simulink model "fullsystem"  (Simulink 8.5)
settings: Solver=ode15s  SolverMode=SingleTasking  StartTime=0.0  StopTime=0.1  RelTol=1e-3  AbsTol=1e-6
undefined symbols (not defined in the file or in its folder): DAB, den, elements, num
libraries: powerlib x43, powerlib_extras x1
(part 1 of 6)
settings Model: Creator=Dr. Lotfifard  LastModifiedBy=PC  ExtModeTrigMode=oneshot  ExtModeArmWhenConnect=off
settings SolverCC: ZeroCrossAlgorithm=Adaptive
settings DataIOCC: LimitDataPoints=off
settings OptimizationCC: BlockReduction=off  BooleanDataType=off
settings DebuggingCC: SaveWithParameterizedLinksMsg=none  SignalResolutionControl=TryResolveAllWithWarning  MultiTaskDSMMsg=warning  MultiTaskCondExecSysMsg=none  FcnCallInpInsideContextMsg=UseLocalSettings
settings HardwareCC: TargetUnknown=on

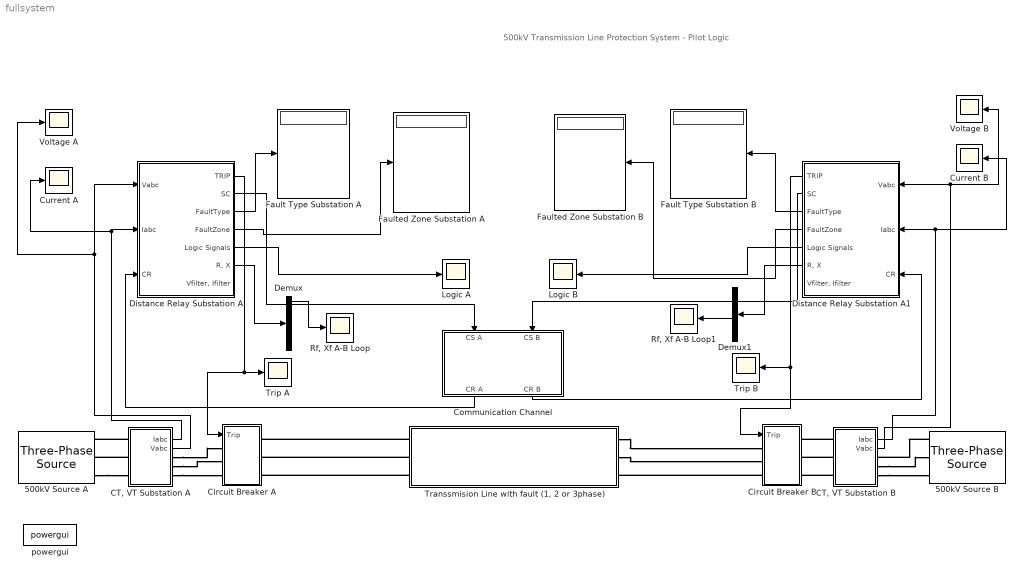
== system fullsystem ==
  note: 500kV Transmission Line Protection System - Pilot Logic
  500kV Source A : powerlib/Electrical Sources/Three-Phase Source  Voltage=500000/sqrt(3)*sqrt(2)  PhaseAngle=0  Frequency=60  InternalConnection=Yg  SpecifyImpedance=off  Resistance=0.724  Inductance=19.2e-3  ShortCircuitLevel=100e6  BaseVoltage=25e3  XRratio=7  BusType=swing  Pref=0  Qref=0  Qmin=-inf  Qmax=inf
  500kV Source B : powerlib/Electrical Sources/Three-Phase Source  Voltage=1.05*500000/sqrt(3)*sqrt(2)  PhaseAngle=10  Frequency=60  InternalConnection=Yg  SpecifyImpedance=off  Resistance=0.724  Inductance=19.2e-3  ShortCircuitLevel=100e6  BaseVoltage=25e3  XRratio=7  BusType=swing  Pref=0  Qref=0  Qmin=-inf  Qmax=inf
  "CT, VT Substation A" : Subsystem  mask{VT=1, CT=1}
      mask prompts: VT "VT ratio"; CT "CT ratio"
  "CT, VT Substation B" : Subsystem  mask{VT=1, CT=1}
      mask prompts: VT "VT ratio"; CT "CT ratio"
  Circuit Breaker A : Subsystem
  Circuit Breaker B : Subsystem
  Communication Channel : Subsystem  mask(Communication channel.){Tdelay=0, failureA=on, failureB=on, err_signal=0}
      mask prompts: Tdelay "Channel delay time [ms]:"; failureA "A to B Communication channel failure."; failureB "B to A Communication Channel failure"; err_signal "Erroneous signal:"
      mask TypeOptions err_signal: 0 | 1
  Current A : Scope
      settings: TickLabels=on  YMin=-8000  YMax=9000
  Current B : Scope
      settings: TickLabels=on  YMin=-8000  YMax=9000  SaveName=ScopeData2
  Demux : Demux  Outputs=6
  Demux1 : Demux  Outputs=6
  Distance Relay Substation A : Subsystem  mask{ZoneImpedance=[90 115 200 250 50], ZoneTime=[0 0.33 1 0.33 0.66], k0m1=0.726, k0a1=-3.69, LineAngle=84, Zstarter=300, Tstarter=0, underV=0.8*500000/sqrt(3)*sqrt(2), PilotLogic='PUTT', fCut=180, fSampling=24*60, WindowSize=24, VoltageRange=480, CurrentRange=480}
      mask prompts: ZoneImpedance "Zone Impedances [Z1 Z2 Z3 Z4 ZR] (Ohm):"; ZoneTime "Zone Times [T1 T2 T3 T4 TR] (s):"; LineAngle "Line Angle:"; Zstarter "Starter Impedance (Ohm):"; Tstarter "Starter Time (s):"; underV "UnderVoltage Threshold (V):"; PilotLogic "Pilot Logic Scheme:"; fCut "fCut (Hz):"; fSampling "fSampling (Hz):"; WindowSize "Window Size (samples):"; VoltageRange "Voltage Range (V):"; CurrentRange "Current Range (A):"
      mask TypeOptions PilotLogic: 'BLOV+TB' | 'PUTT'
  Distance Relay Substation A1 : Subsystem  mask{ZoneImpedance=[90 115 200 250 50], ZoneTime=[0 0.33 1 0.33 0.66], k0m1=0.726, k0a1=-3.69, LineAngle=84, Zstarter=300, Tstarter=0, underV=0.8*1.05*500000/sqrt(3)*sqrt(2), PilotLogic='PUTT', fCut=180, fSampling=24*60, WindowSize=24, VoltageRange=480, CurrentRange=480}
      mask prompts: ZoneImpedance "Zone Impedances [Z1 Z2 Z3 Z4 ZR] (Ohm):"; ZoneTime "Zone Times [T1 T2 T3 T4 TR] (s):"; LineAngle "Line Angle:"; Zstarter "Starter Impedance (Ohm):"; Tstarter "Starter Time (s):"; underV "UnderVoltage Threshold (V):"; PilotLogic "Pilot Logic Scheme:"; fCut "fCut (Hz):"; fSampling "fSampling (Hz):"; WindowSize "Window Size (samples):"; VoltageRange "Voltage Range (V):"; CurrentRange "Current Range (A):"
      mask TypeOptions PilotLogic: 'BLOV+TB' | 'PUTT'
  Fault Type Substation A : Display
  Fault Type Substation B : Display
  Faulted Zone Substation A : Display
  Faulted Zone Substation B : Display
  Logic A : Scope
      settings: SaveName=ScopeData5
  Logic B : Scope
      settings: SaveName=ScopeData4
  "Rf, Xf A-B Loop" : Scope
      settings: YMin=-450  YMax=125
  "Rf, Xf A-B Loop1" : Scope
      settings: SaveName=ScopeData6
  "Transsmision Line with fault (1, 2 or 3phase)" : Subsystem  mask(Teansmission line with fault){ff=60, rr=[0.025485 0.57504], ll=[1.5760e-3 4.5291e-3], cc=[19.1e-9 11.2e-9], length=200, faultLocation=0.5, faultType='A-G', faultR=0.1, faultTime=[0.034 1 2 3 4]}
      mask prompts: ff "Frequency used for R L C specification (Hz)"; rr "Resistance per unit length (Ohm/km) [R1 R0]"; ll "Inductance per unit length (H/km) [L1 L0]"; cc "Capacitance per unit length (F/km) [C1 C0]"; length "Line length (km)"; faultLocation "Fault location (p.u.) <0,1>"; faultType "Fault Type"; faultR "Fault Resistance per Phase (Ohm)"; faultTime "Fault time sequence (s) [C O C O C]"
      mask TypeOptions faultType: 'A-G' | 'A-B' | 'A-B-G' | 'A-B-C' | 'A-B-C-G'
  Trip A : Scope
      settings: SaveName=ScopeData3
  Trip B : Scope
      settings: SaveName=ScopeData7
  Voltage A : Scope
      settings: TickLabels=on  YMin=-400000  YMax=400000
  Voltage B : Scope
      settings: TickLabels=on  SaveName=ScopeData8
  powergui : powerlib/powergui  SimulationMode=Continuous  SolverType=Tustin/Backward Euler (TBE)  SampleTime=0  frequency=60  SPID=off  DisableSnubberDevices=off  DisableRonSwitches=off  DisableVfSwitches=off  SwTol=0  DisplayEquations=off  Interpol=off  methode=off  Ts=0  FunctionMessages=off  echomessages=off  HookPort=off  EnableUseOfTLC=off  x0status=blocks  frequencyindice=60  Pbase=100e6  ErrMax=1e-4  Iterations=50  UnitsV=kV  UnitsW=MW  buscounter=0  RestoreLinks=warning  ResistiveCurrentMeasurement=off  Frange=[0:2:500]  Ylog=off  Xlog=on  ShowGrid=off  save=off  variable=ZData  structure=0  ZoomFFT=on  StartTime=0.0  cycles=1  DisplayStyle=1  fundamental=60  FreqAxis=off  MaxFrequency=1000  frequencyindicesteady=1  RmsSteady=1  display=off
  wires:
  "CT, VT Substation A"/2(Vabc) -> Voltage A/1, Distance Relay Substation A/1(Vabc)
  "CT, VT Substation A"/1(Iabc) -> Current A/1, Distance Relay Substation A/2(Iabc)
  Distance Relay Substation A/3(FaultType) -> Fault Type Substation A/1
  Distance Relay Substation A/4(FaultZone) -> Faulted Zone Substation A/1
  Distance Relay Substation A/1("TRIP ") -> Circuit Breaker A/1(Trip), Trip A/1
  Distance Relay Substation A/5(Logic Signals) -> Logic A/1
  Distance Relay Substation A/6("R, X") -> Demux/1
  Distance Relay Substation A1/3(FaultType) -> Fault Type Substation B/1
  Distance Relay Substation A1/4(FaultZone) -> Faulted Zone Substation B/1
  Distance Relay Substation A1/1("TRIP ") -> Circuit Breaker B/1(Trip), Trip B/1
  Distance Relay Substation A1/6("R, X") -> Demux1/1
  Demux1/4 -> "Rf, Xf A-B Loop1"/1
  Distance Relay Substation A1/5(Logic Signals) -> Logic B/1
  "CT, VT Substation B"/1(Iabc) -> Distance Relay Substation A1/2(Iabc), Current B/1
  "CT, VT Substation B"/2(Vabc) -> Distance Relay Substation A1/1(Vabc), Voltage B/1
  Communication Channel/2(CR B) -> Distance Relay Substation A1/3(CR)
  Distance Relay Substation A1/2(SC) -> Communication Channel/2(CS B)
  Distance Relay Substation A/2(SC) -> Communication Channel/1(CS A)
  Communication Channel/1(CR A) -> Distance Relay Substation A/3(CR)
  Demux/1 -> "Rf, Xf A-B Loop"/1
  connections:
  "CT, VT Substation A"/LConn1 -- 500kV Source A/RConn1
  500kV Source A/RConn3 -- "CT, VT Substation A"/LConn3
  "CT, VT Substation A"/LConn2 -- 500kV Source A/RConn2
  "CT, VT Substation A"/RConn3 -- Circuit Breaker A/LConn3
  "Transsmision Line with fault (1, 2 or 3phase)"/LConn1 -- Circuit Breaker A/RConn1
  "Transsmision Line with fault (1, 2 or 3phase)"/LConn2 -- Circuit Breaker A/RConn2
  "Transsmision Line with fault (1, 2 or 3phase)"/LConn3 -- Circuit Breaker A/RConn3
  Circuit Breaker B/LConn3 -- "Transsmision Line with fault (1, 2 or 3phase)"/RConn3
  "Transsmision Line with fault (1, 2 or 3phase)"/RConn2 -- Circuit Breaker B/LConn2
  "Transsmision Line with fault (1, 2 or 3phase)"/RConn1 -- Circuit Breaker B/LConn1
  "CT, VT Substation B"/LConn1 -- Circuit Breaker B/RConn1
  "CT, VT Substation B"/LConn2 -- Circuit Breaker B/RConn2
  "CT, VT Substation B"/LConn3 -- Circuit Breaker B/RConn3
  500kV Source B/RConn1 -- "CT, VT Substation B"/RConn1
  "CT, VT Substation B"/RConn2 -- 500kV Source B/RConn2
  "CT, VT Substation B"/RConn3 -- 500kV Source B/RConn3
  "CT, VT Substation A"/RConn1 -- Circuit Breaker A/LConn1
  "CT, VT Substation A"/RConn2 -- Circuit Breaker A/LConn2

== system fullsystem/CT, VT Substation A ==
  CT-ratio : Gain  Gain=1/CT  SaturateOnIntegerOverflow=on  OutDataTypeStr=Inherit: Same as input  ParamDataTypeStr=Inherit: Same as input
  Ground : powerlib/Elements/Ground  LConnTagsString=a
  IA : powerlib/Measurements/Current Measurement  PhasorSimulation=off  OutputType=Complex  PSBequivalent=0
  IB1 : powerlib/Measurements/Current Measurement  PhasorSimulation=off  OutputType=Complex  PSBequivalent=0
  IC1 : powerlib/Measurements/Current Measurement  PhasorSimulation=off  OutputType=Complex  PSBequivalent=0
  Mux : Mux  Inputs=3
  Mux1 : Mux  Inputs=3
  VA1 : powerlib/Measurements/Voltage Measurement  PhasorSimulation=off  OutputType=Complex  PSBequivalent=0
  VB1 : powerlib/Measurements/Voltage Measurement  PhasorSimulation=off  OutputType=Complex  PSBequivalent=0
  VC1 : powerlib/Measurements/Voltage Measurement  PhasorSimulation=off  OutputType=Complex  PSBequivalent=0
  VT-ratio : Gain  Gain=1/VT  SaturateOnIntegerOverflow=on  OutDataTypeStr=Inherit: Same as input  ParamDataTypeStr=Inherit: Same as input
  Ain : PMIOPort  Port=1  Side=Left
  Bin : PMIOPort  Port=2  Side=Left
  Cin : PMIOPort  Port=3  Side=Left
  Aout : PMIOPort  Port=4  Side=Right
  Bout : PMIOPort  Port=5  Side=Right
  Cout : PMIOPort  Port=6  Side=Right
  Iabc : Outport
  Vabc : Outport  Port=2
  wires:
  Mux/1 -> CT-ratio/1
  Mux1/1 -> VT-ratio/1
  IA/1 -> Mux/1
  IB1/1 -> Mux/2
  IC1/1 -> Mux/3
  VC1/1 -> Mux1/3
  VB1/1 -> Mux1/2
  VA1/1 -> Mux1/1
  CT-ratio/1 -> Iabc/1
  VT-ratio/1 -> Vabc/1
  connections:
  VC1/LConn2 -- Ground/LConn1 -- VB1/LConn2 -- VA1/LConn2
  Ain/RConn1 -- IA/LConn1 -- VA1/LConn1
  IB1/LConn1 -- Bin/RConn1 -- VB1/LConn1
  IC1/LConn1 -- Cin/RConn1 -- VC1/LConn1
  Cout/RConn1 -- IC1/RConn1
  Aout/RConn1 -- IA/RConn1
  Bout/RConn1 -- IB1/RConn1

== system fullsystem/CT, VT Substation B ==
  CT-ratio : Gain  Gain=1/CT  SaturateOnIntegerOverflow=on  OutDataTypeStr=Inherit: Same as input  ParamDataTypeStr=Inherit: Same as input
  Ground : powerlib/Elements/Ground  LConnTagsString=a
  IA : powerlib/Measurements/Current Measurement  PhasorSimulation=off  OutputType=Complex  PSBequivalent=0
  IB1 : powerlib/Measurements/Current Measurement  PhasorSimulation=off  OutputType=Complex  PSBequivalent=0
  IC1 : powerlib/Measurements/Current Measurement  PhasorSimulation=off  OutputType=Complex  PSBequivalent=0
  Mux : Mux  Inputs=3
  Mux1 : Mux  Inputs=3
  VA1 : powerlib/Measurements/Voltage Measurement  PhasorSimulation=off  OutputType=Complex  PSBequivalent=0
  VB1 : powerlib/Measurements/Voltage Measurement  PhasorSimulation=off  OutputType=Complex  PSBequivalent=0
  VC1 : powerlib/Measurements/Voltage Measurement  PhasorSimulation=off  OutputType=Complex  PSBequivalent=0
  VT-ratio : Gain  Gain=1/VT  SaturateOnIntegerOverflow=on  OutDataTypeStr=Inherit: Same as input  ParamDataTypeStr=Inherit: Same as input
  Ain : PMIOPort  Port=1  Side=Left
  Bin : PMIOPort  Port=2  Side=Left
  Cin : PMIOPort  Port=3  Side=Left
  Aout : PMIOPort  Port=4  Side=Right
  Bout : PMIOPort  Port=5  Side=Right
  Cout : PMIOPort  Port=6  Side=Right
  Iabc : Outport
  Vabc : Outport  Port=2
  wires:
  Mux/1 -> CT-ratio/1
  Mux1/1 -> VT-ratio/1
  IA/1 -> Mux/1
  IB1/1 -> Mux/2
  IC1/1 -> Mux/3
  VC1/1 -> Mux1/3
  VB1/1 -> Mux1/2
  VA1/1 -> Mux1/1
  CT-ratio/1 -> Iabc/1
  VT-ratio/1 -> Vabc/1
  connections:
  VC1/LConn2 -- Ground/LConn1 -- VB1/LConn2 -- VA1/LConn2
  Ain/RConn1 -- IA/LConn1 -- VA1/LConn1
  IB1/LConn1 -- Bin/RConn1 -- VB1/LConn1
  IC1/LConn1 -- Cin/RConn1 -- VC1/LConn1
  Cout/RConn1 -- IC1/RConn1
  Aout/RConn1 -- IA/RConn1
  Bout/RConn1 -- IB1/RConn1

== system fullsystem/Circuit Breaker A ==
  Trip : Inport
  10000 ohms3 : powerlib/Elements/Series RLC Branch  LConnTagsString=__new0  RConnTagsString=__new0  BranchType=R  Resistance=10000  Inductance=1e-3  SetiL0=off  InitialCurrent=0  Capacitance=1e-6  Setx0=off  InitialVoltage=0  Measurements=None
  10000 ohms4 : powerlib/Elements/Series RLC Branch  LConnTagsString=__new0  RConnTagsString=__new0  BranchType=R  Resistance=10000  Inductance=1e-3  SetiL0=off  InitialCurrent=0  Capacitance=1e-6  Setx0=off  InitialVoltage=0  Measurements=None
  10000 ohms5 : powerlib/Elements/Series RLC Branch  LConnTagsString=__new0  RConnTagsString=__new0  BranchType=R  Resistance=10000  Inductance=1e-3  SetiL0=off  InitialCurrent=0  Capacitance=1e-6  Setx0=off  InitialVoltage=0  Measurements=None
  Breaker3 : powerlib/Elements/Breaker  InitialState=0  SwitchingTimes="[ 1/60  5/60 ]"  External=on  BreakerResistance=0.01  SnubberResistance=1e6  SnubberCapacitance=inf  Measurements=None  MoreParameters=off  NoBreakLoop=off
  Breaker4 : powerlib/Elements/Breaker  InitialState=0  SwitchingTimes="[ 1/60  5/60 ]"  External=on  BreakerResistance=0.01  SnubberResistance=1e6  SnubberCapacitance=inf  Measurements=None  MoreParameters=off  NoBreakLoop=off
  Breaker5 : powerlib/Elements/Breaker  InitialState=0  SwitchingTimes="[ 1/60  5/60 ]"  External=on  BreakerResistance=0.01  SnubberResistance=1e6  SnubberCapacitance=inf  Measurements=None  MoreParameters=off  NoBreakLoop=off
  NOT1 : Logic  Operator=NOT  Inputs=1
  Ain : PMIOPort  Port=1  Side=Left
  Aout : PMIOPort  Port=2  Side=Right
  Bin : PMIOPort  Port=3  Side=Right
  Bout : PMIOPort  Port=4  Side=Left
  Cin : PMIOPort  Port=5  Side=Left
  Cout : PMIOPort  Port=6  Side=Right
  wires:
  Trip/1 -> NOT1/1
  NOT1/1 -> Breaker3/1, Breaker4/1, Breaker5/1
  connections:
  10000 ohms3/LConn1 -- Ain/RConn1 -- Breaker3/LConn1
  Aout/RConn1 -- 10000 ohms3/RConn1 -- Breaker3/RConn1
  10000 ohms4/LConn1 -- Bin/RConn1 -- Breaker4/LConn1
  10000 ohms4/RConn1 -- Bout/RConn1 -- Breaker4/RConn1
  10000 ohms5/LConn1 -- Cin/RConn1 -- Breaker5/LConn1
  Cout/RConn1 -- 10000 ohms5/RConn1 -- Breaker5/RConn1

== system fullsystem/Circuit Breaker B ==
  Trip : Inport
  10000 ohms3 : powerlib/Elements/Series RLC Branch  LConnTagsString=__new0  RConnTagsString=__new0  BranchType=R  Resistance=10000  Inductance=1e-3  SetiL0=off  InitialCurrent=0  Capacitance=1e-6  Setx0=off  InitialVoltage=0  Measurements=None
  10000 ohms4 : powerlib/Elements/Series RLC Branch  LConnTagsString=__new0  RConnTagsString=__new0  BranchType=R  Resistance=10000  Inductance=1e-3  SetiL0=off  InitialCurrent=0  Capacitance=1e-6  Setx0=off  InitialVoltage=0  Measurements=None
  10000 ohms5 : powerlib/Elements/Series RLC Branch  LConnTagsString=__new0  RConnTagsString=__new0  BranchType=R  Resistance=10000  Inductance=1e-3  SetiL0=off  InitialCurrent=0  Capacitance=1e-6  Setx0=off  InitialVoltage=0  Measurements=None
  Breaker3 : powerlib/Elements/Breaker  InitialState=0  SwitchingTimes="[ 1/60  5/60 ]"  External=on  BreakerResistance=0.01  SnubberResistance=1e6  SnubberCapacitance=inf  Measurements=None  MoreParameters=off  NoBreakLoop=off
  Breaker4 : powerlib/Elements/Breaker  InitialState=0  SwitchingTimes="[ 1/60  5/60 ]"  External=on  BreakerResistance=0.01  SnubberResistance=1e6  SnubberCapacitance=inf  Measurements=None  MoreParameters=off  NoBreakLoop=off
  Breaker5 : powerlib/Elements/Breaker  InitialState=0  SwitchingTimes="[ 1/60  5/60 ]"  External=on  BreakerResistance=0.01  SnubberResistance=1e6  SnubberCapacitance=inf  Measurements=None  MoreParameters=off  NoBreakLoop=off
  NOT1 : Logic  Operator=NOT  Inputs=1
  Ain : PMIOPort  Port=1  Side=Left
  Aout : PMIOPort  Port=2  Side=Right
  Bin : PMIOPort  Port=3  Side=Right
  Bout : PMIOPort  Port=4  Side=Left
  Cin : PMIOPort  Port=5  Side=Left
  Cout : PMIOPort  Port=6  Side=Right
  wires:
  Trip/1 -> NOT1/1
  NOT1/1 -> Breaker3/1, Breaker4/1, Breaker5/1
  connections:
  10000 ohms3/LConn1 -- Ain/RConn1 -- Breaker3/LConn1
  Aout/RConn1 -- 10000 ohms3/RConn1 -- Breaker3/RConn1
  10000 ohms4/LConn1 -- Bin/RConn1 -- Breaker4/LConn1
  10000 ohms4/RConn1 -- Bout/RConn1 -- Breaker4/RConn1
  10000 ohms5/LConn1 -- Cin/RConn1 -- Breaker5/LConn1
  Cout/RConn1 -- 10000 ohms5/RConn1 -- Breaker5/RConn1

== system fullsystem/Communication Channel ==
  CS A : Inport
  CS B : Inport  Port=2
  " " : Constant  Value=failureA
  "  " : Constant  Value=err_signal-1
  " 1" : Constant  Value=failureB
  Switch : Switch  Threshold=0.5  SaturateOnIntegerOverflow=on  InputSameDT=on
  Switch1 : Switch  Threshold=0.5  SaturateOnIntegerOverflow=on  InputSameDT=on
  delay A->B : TransportDelay  DelayTime=Tdelay/1000+1e-12
  delay B->A : TransportDelay  DelayTime=Tdelay/1000+1e-12
  CR A : Outport  InitialOutput=0
  CR B : Outport  Port=2  InitialOutput=0
  wires:
  Switch/1 -> CR A/1
  CS B/1 -> delay A->B/1
  CS A/1 -> delay B->A/1
  Switch1/1 -> CR B/1
  "  "/1 -> Switch1/1, Switch/1
  delay A->B/1 -> Switch/3
  delay B->A/1 -> Switch1/3
  " "/1 -> Switch1/2
  " 1"/1 -> Switch/2

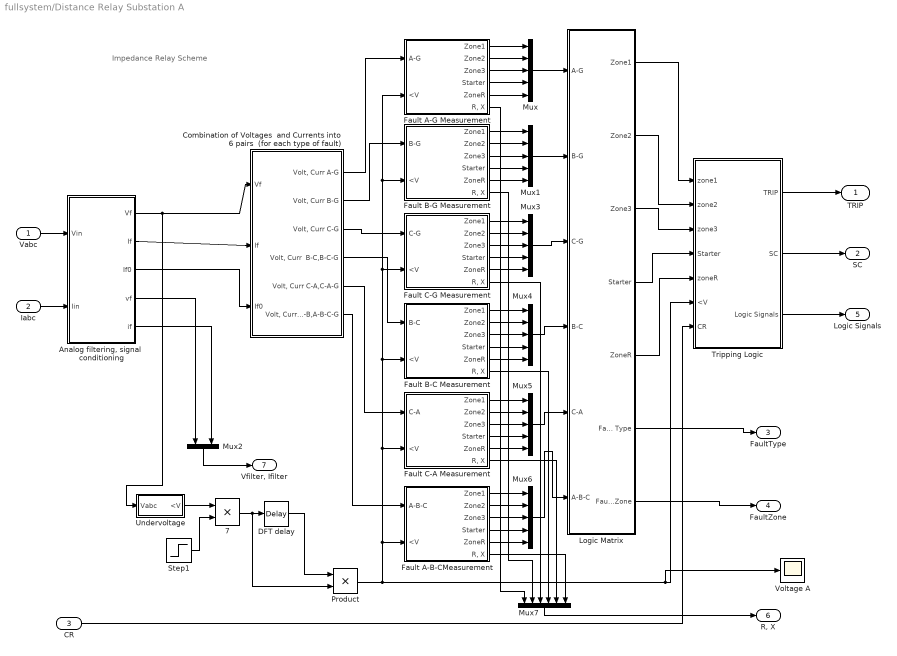
== system fullsystem/Distance Relay Substation A ==
  note: Impedance Relay Scheme
  Vabc : Inport
  Iabc : Inport  Port=2
  CR : Inport  Port=3
  " 7" : Product  RndMeth=Zero
  "Analog filtering, signal  conditioning" : Subsystem
  Combination of Voltages  and Currents into 6 pairs  (for each type of fault) : Subsystem
  DFT delay : TransportDelay  DelayTime=0.017  BufferSize=30720
  Fault A-B-CMeasurement : Subsystem
  Fault A-G Measurement : Subsystem
  Fault B-C Measurement : Subsystem
  Fault B-G Measurement : Subsystem
  Fault C-A Measurement : Subsystem
  Fault C-G Measurement : Subsystem
  Logic Matrix : Subsystem
  Mux{,1,3..6} (6 alike) : Mux  Inputs=5
  Mux2 : Mux  Inputs=2
  Mux7 : Mux  Inputs=6
  Product : Product  RndMeth=Zero
  Step1 : Step  Time=0.017  SampleTime=0
  Tripping Logic : Subsystem
  Undervoltage : Subsystem
  Voltage A : Scope
      settings: TickLabels=on  YMin=-400000  YMax=400000  SaveName=ScopeData9
  "TRIP " : Outport  InitialOutput=0
  SC : Outport  Port=2  InitialOutput=0
  FaultType : Outport  Port=3  InitialOutput=0
  FaultZone : Outport  Port=4  InitialOutput=0
  Logic Signals : Outport  Port=5  InitialOutput=0
  "R, X" : Outport  Port=6  InitialOutput=0
  "Vfilter, Ifilter" : Outport  Port=7  InitialOutput=0
  wires:
  Mux2/1 -> "Vfilter, Ifilter"/1
  Product/1 -> Fault A-B-CMeasurement/2(<V), Fault C-A Measurement/2(<V), Fault B-C Measurement/2(<V), Fault C-G Measurement/2(<V), Fault B-G Measurement/2(<V), Fault A-G Measurement/2(<V), Voltage A/1, Tripping Logic/6(<V)
  Logic Matrix/6(Fault Type) -> FaultType/1
  Tripping Logic/1(TRIP) -> "TRIP "/1
  Logic Matrix/3(" Zone3") -> Tripping Logic/3(zone3)
  Logic Matrix/2(" Zone2") -> Tripping Logic/2(zone2)
  Logic Matrix/1(" Zone1") -> Tripping Logic/1(zone1)
  Mux6/1 -> Logic Matrix/6(A-B-C)
  Mux5/1 -> Logic Matrix/5(C-A)
  Mux4/1 -> Logic Matrix/4(B-C)
  Mux3/1 -> Logic Matrix/3(C-G)
  Mux1/1 -> Logic Matrix/2(B-G)
  Mux/1 -> Logic Matrix/1(A-G)
  Fault B-G Measurement/2(Zone2) -> Mux1/2
  Fault A-G Measurement/4(Starter) -> Mux/4
  Fault A-G Measurement/3(Zone3) -> Mux/3
  Fault A-G Measurement/2(Zone2) -> Mux/2
  Fault A-G Measurement/1(Zone1) -> Mux/1
  DFT delay/1 -> Product/1
  Combination of Voltages  and Currents into 6 pairs  (for each type of fault)/5("Volt, Curr C-A,C-A-G") -> Fault C-A Measurement/1(C-A)
  Combination of Voltages  and Currents into 6 pairs  (for each type of fault)/2("Volt, Curr B-G") -> Fault B-G Measurement/1(B-G)
  "Analog filtering, signal  conditioning"/3(If0) -> Combination of Voltages  and Currents into 6 pairs  (for each type of fault)/3(If0)
  "Analog filtering, signal  conditioning"/2(If) -> Combination of Voltages  and Currents into 6 pairs  (for each type of fault)/2(If)
  "Analog filtering, signal  conditioning"/5(if) -> Mux2/2
  "Analog filtering, signal  conditioning"/4(vf) -> Mux2/1
  "Analog filtering, signal  conditioning"/1(Vf) -> Undervoltage/1("Vabc  "), Combination of Voltages  and Currents into 6 pairs  (for each type of fault)/1(Vf)
  " 7"/1 -> Product/2, DFT delay/1
  Step1/1 -> " 7"/2
  Undervoltage/1(<V) -> " 7"/1
  Combination of Voltages  and Currents into 6 pairs  (for each type of fault)/1("Volt, Curr A-G") -> Fault A-G Measurement/1(A-G)
  Iabc/1 -> "Analog filtering, signal  conditioning"/2(Iin)
  Vabc/1 -> "Analog filtering, signal  conditioning"/1(Vin)
  Fault B-G Measurement/1(Zone1) -> Mux1/1
  Fault B-G Measurement/3(Zone3) -> Mux1/3
  Fault A-G Measurement/5(ZoneR) -> Mux/5
  Fault B-G Measurement/4(Starter) -> Mux1/4
  Fault B-G Measurement/5(ZoneR) -> Mux1/5
  Combination of Voltages  and Currents into 6 pairs  (for each type of fault)/3("Volt, Curr C-G") -> Fault C-G Measurement/1(C-G)
  Fault C-G Measurement/1(Zone1) -> Mux3/1
  Fault C-G Measurement/2(Zone2) -> Mux3/2
  Fault C-G Measurement/3(Zone3) -> Mux3/3
  Fault C-G Measurement/4(Starter) -> Mux3/4
  Fault C-G Measurement/5(ZoneR) -> Mux3/5
  Combination of Voltages  and Currents into 6 pairs  (for each type of fault)/4("Volt, Curr  B-C,B-C-G") -> Fault B-C Measurement/1(B-C)
  Fault B-C Measurement/1(Zone1) -> Mux4/1
  Fault B-C Measurement/2(Zone2) -> Mux4/2
  Fault B-C Measurement/3(Zone3) -> Mux4/3
  Fault B-C Measurement/4(Starter) -> Mux4/4
  Fault B-C Measurement/5(ZoneR) -> Mux4/5
  Fault C-A Measurement/1(Zone1) -> Mux5/1
  Fault C-A Measurement/2(Zone2) -> Mux5/2
  Fault C-A Measurement/3(Zone3) -> Mux5/3
  Fault C-A Measurement/4(Starter) -> Mux5/4
  Fault C-A Measurement/5(ZoneR) -> Mux5/5
  Fault A-B-CMeasurement/1(Zone1) -> Mux6/1
  Fault A-B-CMeasurement/2(Zone2) -> Mux6/2
  Fault A-B-CMeasurement/3(Zone3) -> Mux6/3
  Fault A-B-CMeasurement/4(Starter) -> Mux6/4
  Fault A-B-CMeasurement/5(ZoneR) -> Mux6/5
  Combination of Voltages  and Currents into 6 pairs  (for each type of fault)/6("Volt, Curr A-B,A-B-C-G") -> Fault A-B-CMeasurement/1(A-B-C)
  Mux7/1 -> "R, X"/1
  Fault A-B-CMeasurement/6("R, X") -> Mux7/6
  Fault C-A Measurement/6("R, X") -> Mux7/5
  Fault B-C Measurement/6("R, X") -> Mux7/4
  Fault C-G Measurement/6("R, X") -> Mux7/3
  Fault B-G Measurement/6("R, X") -> Mux7/2
  Fault A-G Measurement/6("R, X") -> Mux7/1
  Logic Matrix/7(Fault Zone) -> FaultZone/1
  Tripping Logic/2(SC) -> SC/1
  Tripping Logic/3(Logic Signals) -> Logic Signals/1
  CR/1 -> Tripping Logic/7(CR)
  Logic Matrix/4(" Starter") -> Tripping Logic/4(Starter)
  Logic Matrix/5(" ZoneR") -> Tripping Logic/5(zoneR)

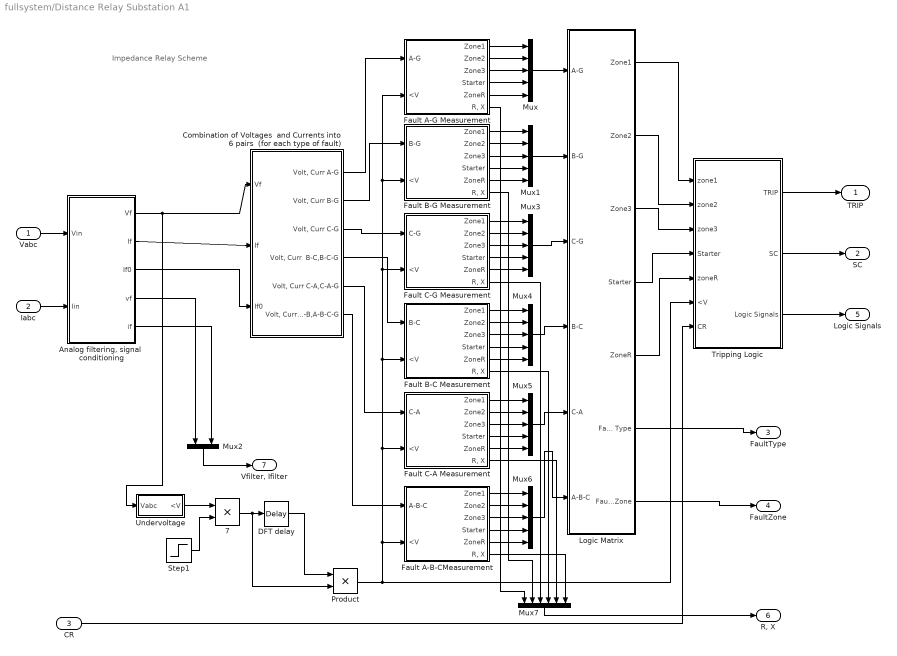
== system fullsystem/Distance Relay Substation A1 ==
  note: Impedance Relay Scheme
  Vabc : Inport
  Iabc : Inport  Port=2
  CR : Inport  Port=3
  " 7" : Product  RndMeth=Zero
  "Analog filtering, signal  conditioning" : Subsystem
  Combination of Voltages  and Currents into 6 pairs  (for each type of fault) : Subsystem
  DFT delay : TransportDelay  DelayTime=0.017  BufferSize=30720
  Fault A-B-CMeasurement : Subsystem
  Fault A-G Measurement : Subsystem
  Fault B-C Measurement : Subsystem
  Fault B-G Measurement : Subsystem
  Fault C-A Measurement : Subsystem
  Fault C-G Measurement : Subsystem
  Logic Matrix : Subsystem
  Mux{,1,3..6} (6 alike) : Mux  Inputs=5
  Mux2 : Mux  Inputs=2
  Mux7 : Mux  Inputs=6
  Product : Product  RndMeth=Zero
  Step1 : Step  Time=0.017  SampleTime=0
  Tripping Logic : Subsystem
  Undervoltage : Subsystem
  "TRIP " : Outport  InitialOutput=0
  SC : Outport  Port=2  InitialOutput=0
  FaultType : Outport  Port=3  InitialOutput=0
  FaultZone : Outport  Port=4  InitialOutput=0
  Logic Signals : Outport  Port=5  InitialOutput=0
  "R, X" : Outport  Port=6  InitialOutput=0
  "Vfilter, Ifilter" : Outport  Port=7  InitialOutput=0
  wires:
  Mux2/1 -> "Vfilter, Ifilter"/1
  Product/1 -> Fault A-B-CMeasurement/2(<V), Fault C-A Measurement/2(<V), Fault B-C Measurement/2(<V), Fault C-G Measurement/2(<V), Fault B-G Measurement/2(<V), Fault A-G Measurement/2(<V), Tripping Logic/6(<V)
  Logic Matrix/6(Fault Type) -> FaultType/1
  Tripping Logic/1(TRIP) -> "TRIP "/1
  Logic Matrix/3(" Zone3") -> Tripping Logic/3(zone3)
  Logic Matrix/2(" Zone2") -> Tripping Logic/2(zone2)
  Logic Matrix/1(" Zone1") -> Tripping Logic/1(zone1)
  Mux6/1 -> Logic Matrix/6(A-B-C)
  Mux5/1 -> Logic Matrix/5(C-A)
  Mux4/1 -> Logic Matrix/4(B-C)
  Mux3/1 -> Logic Matrix/3(C-G)
  Mux1/1 -> Logic Matrix/2(B-G)
  Mux/1 -> Logic Matrix/1(A-G)
  Fault B-G Measurement/2(Zone2) -> Mux1/2
  Fault A-G Measurement/4(Starter) -> Mux/4
  Fault A-G Measurement/3(Zone3) -> Mux/3
  Fault A-G Measurement/2(Zone2) -> Mux/2
  Fault A-G Measurement/1(Zone1) -> Mux/1
  DFT delay/1 -> Product/1
  Combination of Voltages  and Currents into 6 pairs  (for each type of fault)/5("Volt, Curr C-A,C-A-G") -> Fault C-A Measurement/1(C-A)
  Combination of Voltages  and Currents into 6 pairs  (for each type of fault)/2("Volt, Curr B-G") -> Fault B-G Measurement/1(B-G)
  "Analog filtering, signal  conditioning"/3(If0) -> Combination of Voltages  and Currents into 6 pairs  (for each type of fault)/3(If0)
  "Analog filtering, signal  conditioning"/2(If) -> Combination of Voltages  and Currents into 6 pairs  (for each type of fault)/2(If)
  "Analog filtering, signal  conditioning"/5(if) -> Mux2/2
  "Analog filtering, signal  conditioning"/4(vf) -> Mux2/1
  "Analog filtering, signal  conditioning"/1(Vf) -> Undervoltage/1("Vabc  "), Combination of Voltages  and Currents into 6 pairs  (for each type of fault)/1(Vf)
  " 7"/1 -> Product/2, DFT delay/1
  Step1/1 -> " 7"/2
  Undervoltage/1(<V) -> " 7"/1
  Combination of Voltages  and Currents into 6 pairs  (for each type of fault)/1("Volt, Curr A-G") -> Fault A-G Measurement/1(A-G)
  Iabc/1 -> "Analog filtering, signal  conditioning"/2(Iin)
  Vabc/1 -> "Analog filtering, signal  conditioning"/1(Vin)
  Fault B-G Measurement/1(Zone1) -> Mux1/1
  Fault B-G Measurement/3(Zone3) -> Mux1/3
  Fault A-G Measurement/5(ZoneR) -> Mux/5
  Fault B-G Measurement/4(Starter) -> Mux1/4
  Fault B-G Measurement/5(ZoneR) -> Mux1/5
  Combination of Voltages  and Currents into 6 pairs  (for each type of fault)/3("Volt, Curr C-G") -> Fault C-G Measurement/1(C-G)
  Fault C-G Measurement/1(Zone1) -> Mux3/1
  Fault C-G Measurement/2(Zone2) -> Mux3/2
  Fault C-G Measurement/3(Zone3) -> Mux3/3
  Fault C-G Measurement/4(Starter) -> Mux3/4
  Fault C-G Measurement/5(ZoneR) -> Mux3/5
  Combination of Voltages  and Currents into 6 pairs  (for each type of fault)/4("Volt, Curr  B-C,B-C-G") -> Fault B-C Measurement/1(B-C)
  Fault B-C Measurement/1(Zone1) -> Mux4/1
  Fault B-C Measurement/2(Zone2) -> Mux4/2
  Fault B-C Measurement/3(Zone3) -> Mux4/3
  Fault B-C Measurement/4(Starter) -> Mux4/4
  Fault B-C Measurement/5(ZoneR) -> Mux4/5
  Fault C-A Measurement/1(Zone1) -> Mux5/1
  Fault C-A Measurement/2(Zone2) -> Mux5/2
  Fault C-A Measurement/3(Zone3) -> Mux5/3
  Fault C-A Measurement/4(Starter) -> Mux5/4
  Fault C-A Measurement/5(ZoneR) -> Mux5/5
  Fault A-B-CMeasurement/1(Zone1) -> Mux6/1
  Fault A-B-CMeasurement/2(Zone2) -> Mux6/2
  Fault A-B-CMeasurement/3(Zone3) -> Mux6/3
  Fault A-B-CMeasurement/4(Starter) -> Mux6/4
  Fault A-B-CMeasurement/5(ZoneR) -> Mux6/5
  Combination of Voltages  and Currents into 6 pairs  (for each type of fault)/6("Volt, Curr A-B,A-B-C-G") -> Fault A-B-CMeasurement/1(A-B-C)
  Mux7/1 -> "R, X"/1
  Fault A-B-CMeasurement/6("R, X") -> Mux7/6
  Fault C-A Measurement/6("R, X") -> Mux7/5
  Fault B-C Measurement/6("R, X") -> Mux7/4
  Fault C-G Measurement/6("R, X") -> Mux7/3
  Fault B-G Measurement/6("R, X") -> Mux7/2
  Fault A-G Measurement/6("R, X") -> Mux7/1
  Logic Matrix/7(Fault Zone) -> FaultZone/1
  Tripping Logic/2(SC) -> SC/1
  Tripping Logic/3(Logic Signals) -> Logic Signals/1
  CR/1 -> Tripping Logic/7(CR)
  Logic Matrix/4(" Starter") -> Tripping Logic/4(Starter)
  Logic Matrix/5(" ZoneR") -> Tripping Logic/5(zoneR)

== system fullsystem/Transsmision Line with fault (1, 2 or 3phase) ==
  Fault Selector : Subsystem
  Fault1 : Subsystem
  Line1 : powerlib/Elements/Distributed Parameters Line  Phases=3  Frequency=ff  Resistance=rr  Inductance=ll  Capacitance=cc  Length=length*(faultLocation+0.0005)  x1=[0 1.53266796670346e-009 -40255.985134743 -39683.0380465592;2.86312968195295e-005 1.53189939694959e-009 -39825.3198862797 -40115.2308198371;5.7262593639059e-005 1.53095235510765e-009 -39390.0148370482 -40542.7500166237;8.58938904585885e-005 1.52982695151157e-009 -38950.120701737 -40965.5458293116;0.000114525187278118 1.52852331727516e-009 -38505.688729681 -41383.5690005856;0.000143156484097647 1.52704160427675e-009 -38056.77069889 -41796.7708291612]  x2=[0 1.55925131848491e-009 -40620.0878760363 -39910.0233219334;2.86312968195295e-005 1.55881129165316e-009 -40186.9514443784 -40346.1328285791;5.7262593639059e-005 1.55818965739555e-009 -39749.1330805045 -40777.5418577741;8.58938904585885e-005 1.55738648813482e-009 -39306.6837919141 -41204.2001487306;0.000114525187278118 1.55640187744325e-009 -38859.6551256268 -41626.0579941401;0.000143156484097647 1.55523594003171e-009 -38408.0991621773 -42043.0662459641]  x3=[0 2.01885457122014e-012 -163.089263474603 -105.450555147554;2.86312968195295e-005 2.03239610658583e-012 -161.941578955542 -107.204722130146;5.7262593639059e-005 2.04570086009907e-012 -160.775027628515 -108.946399356132;8.58938904585885e-005 2.05876728170564e-012 -159.589745401176 -110.675383913513;0.000114525187278118 2.07159384911787e-012 -158.385870363398 -112.391474369031;0.000143156484097647 2.08417906799204e-012 -157.163542771187 -114.094470791643]  x4=[0 2.64131154335596e-012 -123.841881809461 -165.416317671308;2.86312968195295e-005 2.63470626197041e-012 -122.049240966749 -166.743373545949;5.7262593639059e-005 2.62779402731559e-012 -120.242380924704 -168.051003185349;8.58938904585885e-005 2.62057564469306e-012 -118.42151218937 -169.339054245695;0.000114525187278118 2.61305195507176e-012 -116.58684689886 -170.607376664157;0.000143156484097647 2.60522383499005e-012 -114.738598798635 -171.855822676363]  x5=0.000143156484097647  V1=[1.023e-09 5.653e+04 5.653e+04;377 377 377;-0.6096 -0.9539 -2.525]  V2=[1.009e-09 5.763e+04 5.763e+04;377 377 377;-0.5917 -0.9614 -2.532]  I1=[1.529e-12 193 193;377 377 377;-0.6847 -1.158 -2.729]  I2=[1.505e-12 205.7 205.7;377 377 377;-0.9069 -0.9704 -2.541]  nHarmo=1  Measurements=None
  Line2 : powerlib/Elements/Distributed Parameters Line  Phases=3  Frequency=ff  Resistance=rr  Inductance=ll  Capacitance=cc  Length=length*(1-faultLocation-0.0005)  x1=[0 1.43137261755031e-009 -51373.762200412 -24567.0115803634;0.000256257228747928 1.48443013216827e-009 -48764.5687185778 -29407.7938360784;0.000512514457495856 1.52364444798437e-009 -45700.6164679546 -33974.3308258324;0.000768771686243784 1.54864986805002e-009 -42210.4786357914 -38224.0368610064;0.00102502891499171 1.55921320186769e-009 -38326.7028447818 -42117.2808911256;0.00128128614373964 1.55523594003171e-009 -34085.5076270153 -45617.7560871077]  x2=[0 1.5552865834267e-009 -50810.114798948 -24266.9121672487;0.000256257228747928 1.62275226289842e-009 -48232.4960307204 -29054.7262706394;0.000512514457495856 1.67508480697045e-009 -45205.080389744 -33571.5876742822;0.000768771686243784 1.71179618336988e-009 -41756.1003375311 -37775.3739441089;0.00102502891499171 1.73254403655516e-009 -37917.719675861 -41626.8822589206;0.00128128614373964 1.73713488038629e-009 -33725.7336000921 -45090.195000142]  x3=[0 1.4523601474402e-012 -189.596238125285 -56.3258357388615;0.000256257228747928 1.62464711268222e-012 -183.279195992341 -74.3509892290754;0.000512514457495856 1.78178327191703e-012 -175.252965739737 -91.6827752763165;0.000768771686243784 1.92230323647857e-012 -165.592396764968 -108.159564609767;0.00102502891499171 2.04489657365404e-012 -154.387579651591 -123.627701314326;0.00128128614373964 2.14842002725272e-012 -141.743006020653 -137.942935763923]  x4=[0 2.19293673092143e-012 -193.598935066748 -45.2078125315412;0.000256257228747928 2.29222269793401e-012 -188.335634767859 -63.6708932672806;0.000512514457495856 2.37013231733818e-012 -181.315992033535 -81.540204842525;0.000768771686243784 2.42593903533621e-012 -172.605469230635 -98.64910523942;0.00102502891499171 2.45912242090544e-012 -162.285297193952 -114.838043729142;0.00128128614373964 2.46937301912888e-012 -150.451717700097 -129.956048777869]  x5=0.00128128614373964  V1=[1.009e-09 5.763e+04 5.763e+04;377 377 377;-0.5911 -0.961 -2.532]  V2=[1.016e-09 5.63e+04 5.63e+04;377 377 377;-0.6002 -0.9605 -2.531]  I1=[1.352e-12 198.8 198.8;377 377 377;-0.8534 -0.9517 -2.522]  I2=[1.642e-12 199.8 199.8;377 377 377;-0.6541 -1.176 -2.747]  nHarmo=1  Measurements=None
  Timer : powerlib_extras/Control  Blocks/Timer  t=[0 faultTime]  e=[0 1 0 1 0 1]
  Ain : PMIOPort  Port=1  Side=Left
  Bin1 : PMIOPort  Port=2  Side=Left
  Cin : PMIOPort  Port=3  Side=Left
  Aout : PMIOPort  Port=4  Side=Right
  Bout : PMIOPort  Port=5  Side=Right
  Cout : PMIOPort  Port=6  Side=Right
  wires:
  Timer/1 -> Fault1/5(Tfault)
  Fault Selector/1(faultA) -> Fault1/1(faultA)
  Fault Selector/2(faultB) -> Fault1/2(faultB)
  Fault Selector/3(faultC) -> Fault1/3(faultC)
  Fault Selector/4(faultR) -> Fault1/4(faultG)
  connections:
  Fault1/LConn1 -- Line2/LConn1 -- Line1/RConn1
  Fault1/LConn2 -- Line1/RConn2 -- Line2/LConn2
  Fault1/LConn3 -- Line2/LConn3 -- Line1/RConn3
  Cin/RConn1 -- Line1/LConn3
  Line1/LConn2 -- Bin1/RConn1
  Line2/RConn3 -- Cout/RConn1
  Ain/RConn1 -- Line1/LConn1
  Line2/RConn2 -- Bout/RConn1
  Line2/RConn1 -- Aout/RConn1

== system fullsystem/Distance Relay Substation A/Analog filtering, signal  conditioning ==
  note: Acquisition Block- analog filtering,
      | signal conditioning, sampling.
  Vin : Inport
  Iin : Inport  Port=2
  CURRENTS : Subsystem
  Mux{1..4} (4 alike) : Mux  Inputs=3
  VOLTAGES : Subsystem
  Vf : Outport  InitialOutput=0
  If : Outport  Port=2  InitialOutput=0
  If0 : Outport  Port=3  InitialOutput=0
  vf : Outport  Port=4  InitialOutput=0
  if : Outport  Port=5  InitialOutput=0
  wires:
  CURRENTS/4(k0I0f) -> If0/1
  Mux4/1 -> if/1
  Mux3/1 -> If/1
  CURRENTS/7(icf) -> Mux4/3
  CURRENTS/6(ibf) -> Mux4/2
  CURRENTS/5(iaf) -> Mux4/1
  CURRENTS/3(ICf) -> Mux3/3
  CURRENTS/2(IBf) -> Mux3/2
  CURRENTS/1(IAf) -> Mux3/1
  Iin/1 -> CURRENTS/1(Iabc)
  Mux2/1 -> vf/1
  VOLTAGES/6(vcf) -> Mux2/3
  VOLTAGES/5(vbf) -> Mux2/2
  VOLTAGES/4(vaf) -> Mux2/1
  VOLTAGES/3(VCf) -> Mux1/3
  VOLTAGES/2(VBf) -> Mux1/2
  VOLTAGES/1(VAf) -> Mux1/1
  Vin/1 -> VOLTAGES/1(Vabc)
  Mux1/1 -> Vf/1

== system fullsystem/Distance Relay Substation A/Combination of Voltages  and Currents into 6 pairs  (for each type of fault) ==
  note: Voltage and current combination block
  Vf : Inport
  If : Inport  Port=2
  If0 : Inport  Port=3
  "Currents Ia, Ib, Ic, kIo" : Demux  Outputs=3
  Ia+kIo : Sum  SaturateOnIntegerOverflow=on  InputSameDT=on  OutDataTypeStr=Inherit: Same as first input
  Ia-Ib : Sum  Inputs=+-  SaturateOnIntegerOverflow=on  InputSameDT=on  OutDataTypeStr=Inherit: Same as first input
  Ib+kIo : Sum  SaturateOnIntegerOverflow=on  InputSameDT=on  OutDataTypeStr=Inherit: Same as first input
  Ib-Ic : Sum  Inputs=+-  SaturateOnIntegerOverflow=on  InputSameDT=on  OutDataTypeStr=Inherit: Same as first input
  Ic+kIo : Sum  SaturateOnIntegerOverflow=on  InputSameDT=on  OutDataTypeStr=Inherit: Same as first input
  Ic-Ia : Sum  Inputs=+-  SaturateOnIntegerOverflow=on  InputSameDT=on  OutDataTypeStr=Inherit: Same as first input
  Mux{10..15} (6 alike) : Mux  Inputs=2
  Va-Vb : Sum  Inputs=+-  SaturateOnIntegerOverflow=on  InputSameDT=on  OutDataTypeStr=Inherit: Same as first input
  Vb-Vc : Sum  Inputs=+-  SaturateOnIntegerOverflow=on  InputSameDT=on  OutDataTypeStr=Inherit: Same as first input
  Vc-Va : Sum  Inputs=+-  SaturateOnIntegerOverflow=on  InputSameDT=on  OutDataTypeStr=Inherit: Same as first input
  "Voltages Va,Vb, Vc" : Demux  Outputs=3
  "Volt, Curr A-G" : Outport  InitialOutput=0
  "Volt, Curr B-G" : Outport  Port=2  InitialOutput=0
  "Volt, Curr C-G" : Outport  Port=3  InitialOutput=0
  "Volt, Curr  B-C,B-C-G" : Outport  Port=4  InitialOutput=0
  "Volt, Curr C-A,C-A-G" : Outport  Port=5  InitialOutput=0
  "Volt, Curr A-B,A-B-C-G" : Outport  Port=6  InitialOutput=0
  wires:
  If0/1 -> Ib+kIo/2, Ia+kIo/2, Ic+kIo/2
  Mux13/1 -> "Volt, Curr  B-C,B-C-G"/1
  Vb-Vc/1 -> Mux13/1
  Ib-Ic/1 -> Mux13/2
  Mux12/1 -> "Volt, Curr C-G"/1
  Ic+kIo/1 -> Mux12/2
  If/1 -> "Currents Ia, Ib, Ic, kIo"/1
  "Voltages Va,Vb, Vc"/3 -> Vc-Va/1, Vb-Vc/2, Mux12/1
  "Voltages Va,Vb, Vc"/2 -> Vb-Vc/1, Mux11/1, Va-Vb/2
  "Voltages Va,Vb, Vc"/1 -> Va-Vb/1, Mux10/1, Vc-Va/2
  Vf/1 -> "Voltages Va,Vb, Vc"/1
  Mux15/1 -> "Volt, Curr A-B,A-B-C-G"/1
  Mux14/1 -> "Volt, Curr C-A,C-A-G"/1
  Vc-Va/1 -> Mux14/1
  Mux11/1 -> "Volt, Curr B-G"/1
  Mux10/1 -> "Volt, Curr A-G"/1
  Ia+kIo/1 -> Mux10/2
  Ib+kIo/1 -> Mux11/2
  Ic-Ia/1 -> Mux14/2
  Va-Vb/1 -> Mux15/1
  Ia-Ib/1 -> Mux15/2
  "Currents Ia, Ib, Ic, kIo"/2 -> Ia-Ib/2, Ib-Ic/1, Ib+kIo/1
  "Currents Ia, Ib, Ic, kIo"/3 -> Ic-Ia/1, Ib-Ic/2, Ic+kIo/1
  "Currents Ia, Ib, Ic, kIo"/1 -> Ia-Ib/1, Ic-Ia/2, Ia+kIo/1

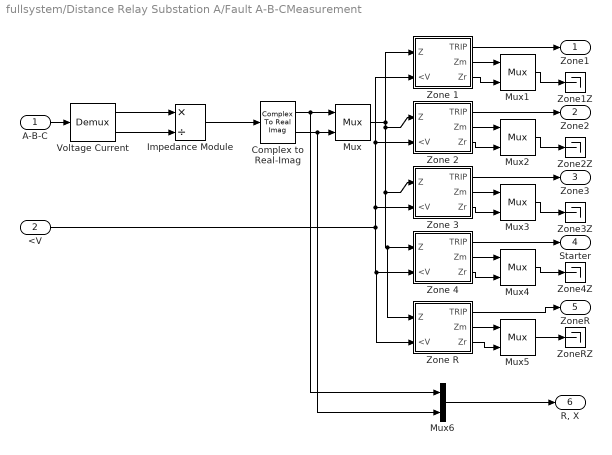
== system fullsystem/Distance Relay Substation A/Fault A-B-CMeasurement ==
  A-B-C : Inport
  <V : Inport  Port=2
  Complex to Real-Imag : ComplexToRealImag
  Impedance Module : Product  Inputs=*/  SaturateOnIntegerOverflow=on  RndMeth=Zero  InputSameDT=on  OutDataTypeStr=Inherit: Same as first input
  Mux{,1..6} (7 alike) : Mux  Inputs=2
  Voltage Current : Demux  Outputs=2
  Zone 1 : Subsystem  mask(Zone){Xr=ZoneImpedance(1)*sin(LineAngle*pi/180), Rr=ZoneImpedance(1)*cos(LineAngle*pi/180), Td=ZoneTime(1)}
      mask prompts: Xr "Reactance reach [ohm]"; Rr "Resistance reach [ohm]"; Td "Time delay [s]"
  Zone 2 : Subsystem  mask(Zone){Xr=ZoneImpedance(2)*sin(LineAngle*pi/180), Rr=ZoneImpedance(2)*cos(LineAngle*pi/180), Td=ZoneTime(2)}
      mask prompts: Xr "Reactance reach [ohm]"; Rr "Resistance reach [ohm]"; Td "Time delay [s]"
  Zone 3 : Subsystem  mask(Zone){Xr=ZoneImpedance(3)*sin(LineAngle*pi/180), Rr=ZoneImpedance(3)*cos(LineAngle*pi/180), Td=ZoneTime(3)}
      mask prompts: Xr "Reactance reach [ohm]"; Rr "Resistance reach [ohm]"; Td "Time delay [s]"
  Zone 4 : Subsystem  mask(Zone){Xr=ZoneImpedance(4)*sin(LineAngle*pi/180), Rr=ZoneImpedance(4)*cos(LineAngle*pi/180), Td=ZoneTime(4)}
      mask prompts: Xr "Reactance reach [ohm]"; Rr "Resistance reach [ohm]"; Td "Time delay [s]"
  Zone R : Subsystem  mask(Zone){Xr=ZoneImpedance(5)*sin(LineAngle*pi/180), Rr=ZoneImpedance(5)*cos(LineAngle*pi/180), Td=ZoneTime(5)}
      mask prompts: Xr "Reactance reach [ohm]"; Rr "Resistance reach [ohm]"; Td "Time delay [s]"
  Zone1Z : Terminator
  Zone2Z : Terminator
  Zone3Z : Terminator
  Zone4Z : Terminator
  ZoneRZ : Terminator
  Zone1 : Outport  InitialOutput=0
  Zone2 : Outport  Port=2  InitialOutput=0
  Zone3 : Outport  Port=3  InitialOutput=0
  Starter : Outport  Port=4  InitialOutput=0
  ZoneR : Outport  Port=5  InitialOutput=0
  "R, X" : Outport  Port=6  InitialOutput=0
  wires:
  Voltage Current/2 -> Impedance Module/2
  Voltage Current/1 -> Impedance Module/1
  Impedance Module/1 -> Complex to Real-Imag/1
  Mux4/1 -> Zone4Z/1
  Mux3/1 -> Zone3Z/1
  Mux2/1 -> Zone2Z/1
  Mux1/1 -> Zone1Z/1
  <V/1 -> Zone R/2(<V), Zone 4/2(<V), Zone 3/2(<V), Zone 2/2(<V), Zone 1/2(<V)
  Complex to Real-Imag/2 -> Mux6/2, Mux/2
  Complex to Real-Imag/1 -> Mux6/1, Mux/1
  Zone 4/1(TRIP) -> Starter/1
  Zone 3/1(TRIP) -> Zone3/1
  Zone 2/1(TRIP) -> Zone2/1
  Zone 4/3(Zr) -> Mux4/2
  Zone 4/2(Zm) -> Mux4/1
  Zone 3/3(Zr) -> Mux3/2
  Zone 3/2(Zm) -> Mux3/1
  Zone 2/3(Zr) -> Mux2/2
  Zone 2/2(Zm) -> Mux2/1
  Zone 1/3(Zr) -> Mux1/2
  Zone 1/2(Zm) -> Mux1/1
  Zone 1/1(TRIP) -> Zone1/1
  Mux/1 -> Zone 2/1(Z), Zone R/1(Z), Zone 4/1(Z), Zone 3/1(Z), Zone 1/1(Z)
  A-B-C/1 -> Voltage Current/1
  Zone R/2(Zm) -> Mux5/1
  Zone R/3(Zr) -> Mux5/2
  Mux5/1 -> ZoneRZ/1
  Zone R/1(TRIP) -> ZoneR/1
  Mux6/1 -> "R, X"/1

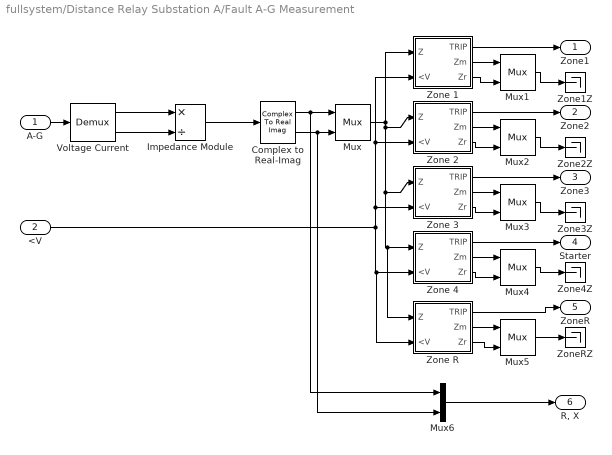
== system fullsystem/Distance Relay Substation A/Fault A-G Measurement ==
  A-G : Inport
  <V : Inport  Port=2
  Complex to Real-Imag : ComplexToRealImag
  Impedance Module : Product  Inputs=*/  SaturateOnIntegerOverflow=on  RndMeth=Zero  InputSameDT=on  OutDataTypeStr=Inherit: Same as first input
  Mux{,1..6} (7 alike) : Mux  Inputs=2
  Voltage Current : Demux  Outputs=2
  Zone 1 : Subsystem  mask(Zone){Xr=ZoneImpedance(1)*sin(LineAngle*pi/180), Rr=ZoneImpedance(1)*cos(LineAngle*pi/180), Td=ZoneTime(1)}
      mask prompts: Xr "Reactance reach [ohm]"; Rr "Resistance reach [ohm]"; Td "Time delay [s]"
  Zone 2 : Subsystem  mask(Zone){Xr=ZoneImpedance(2)*sin(LineAngle*pi/180), Rr=ZoneImpedance(2)*cos(LineAngle*pi/180), Td=ZoneTime(2)}
      mask prompts: Xr "Reactance reach [ohm]"; Rr "Resistance reach [ohm]"; Td "Time delay [s]"
  Zone 3 : Subsystem  mask(Zone){Xr=ZoneImpedance(3)*sin(LineAngle*pi/180), Rr=ZoneImpedance(3)*cos(LineAngle*pi/180), Td=ZoneTime(3)}
      mask prompts: Xr "Reactance reach [ohm]"; Rr "Resistance reach [ohm]"; Td "Time delay [s]"
  Zone 4 : Subsystem  mask(Zone){Xr=ZoneImpedance(4)*sin(LineAngle*pi/180), Rr=ZoneImpedance(4)*cos(LineAngle*pi/180), Td=ZoneTime(4)}
      mask prompts: Xr "Reactance reach [ohm]"; Rr "Resistance reach [ohm]"; Td "Time delay [s]"
  Zone R : Subsystem  mask(Zone){Xr=ZoneImpedance(5)*sin(LineAngle*pi/180), Rr=ZoneImpedance(5)*cos(LineAngle*pi/180), Td=ZoneTime(5)}
      mask prompts: Xr "Reactance reach [ohm]"; Rr "Resistance reach [ohm]"; Td "Time delay [s]"
  Zone1Z : Terminator
  Zone2Z : Terminator
  Zone3Z : Terminator
  Zone4Z : Terminator
  ZoneRZ : Terminator
  Zone1 : Outport  InitialOutput=0
  Zone2 : Outport  Port=2  InitialOutput=0
  Zone3 : Outport  Port=3  InitialOutput=0
  Starter : Outport  Port=4  InitialOutput=0
  ZoneR : Outport  Port=5  InitialOutput=0
  "R, X" : Outport  Port=6  InitialOutput=0
  wires:
  Voltage Current/2 -> Impedance Module/2
  Voltage Current/1 -> Impedance Module/1
  Impedance Module/1 -> Complex to Real-Imag/1
  Mux4/1 -> Zone4Z/1
  Mux3/1 -> Zone3Z/1
  Mux2/1 -> Zone2Z/1
  Mux1/1 -> Zone1Z/1
  <V/1 -> Zone R/2(<V), Zone 4/2(<V), Zone 3/2(<V), Zone 2/2(<V), Zone 1/2(<V)
  Complex to Real-Imag/2 -> Mux6/2, Mux/2
  Complex to Real-Imag/1 -> Mux6/1, Mux/1
  Zone 4/1(TRIP) -> Starter/1
  Zone 3/1(TRIP) -> Zone3/1
  Zone 2/1(TRIP) -> Zone2/1
  Zone 4/3(Zr) -> Mux4/2
  Zone 4/2(Zm) -> Mux4/1
  Zone 3/3(Zr) -> Mux3/2
  Zone 3/2(Zm) -> Mux3/1
  Zone 2/3(Zr) -> Mux2/2
  Zone 2/2(Zm) -> Mux2/1
  Zone 1/3(Zr) -> Mux1/2
  Zone 1/2(Zm) -> Mux1/1
  Zone 1/1(TRIP) -> Zone1/1
  Mux/1 -> Zone 2/1(Z), Zone R/1(Z), Zone 4/1(Z), Zone 3/1(Z), Zone 1/1(Z)
  A-G/1 -> Voltage Current/1
  Zone R/2(Zm) -> Mux5/1
  Zone R/3(Zr) -> Mux5/2
  Mux5/1 -> ZoneRZ/1
  Zone R/1(TRIP) -> ZoneR/1
  Mux6/1 -> "R, X"/1

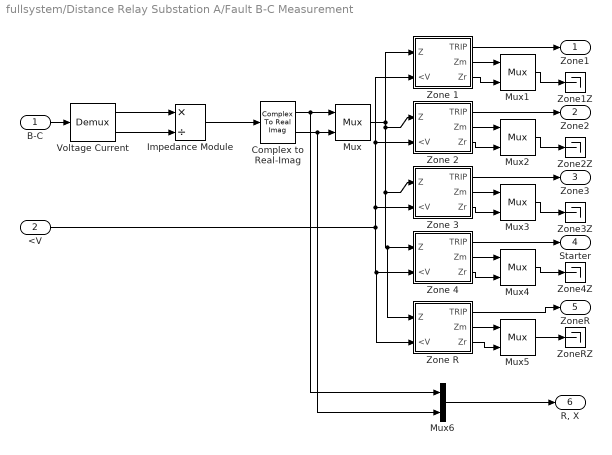
== system fullsystem/Distance Relay Substation A/Fault B-C Measurement ==
  B-C : Inport
  <V : Inport  Port=2
  Complex to Real-Imag : ComplexToRealImag
  Impedance Module : Product  Inputs=*/  SaturateOnIntegerOverflow=on  RndMeth=Zero  InputSameDT=on  OutDataTypeStr=Inherit: Same as first input
  Mux{,1..6} (7 alike) : Mux  Inputs=2
  Voltage Current : Demux  Outputs=2
  Zone 1 : Subsystem  mask(Zone){Xr=ZoneImpedance(1)*sin(LineAngle*pi/180), Rr=ZoneImpedance(1)*cos(LineAngle*pi/180), Td=ZoneTime(1)}
      mask prompts: Xr "Reactance reach [ohm]"; Rr "Resistance reach [ohm]"; Td "Time delay [s]"
  Zone 2 : Subsystem  mask(Zone){Xr=ZoneImpedance(2)*sin(LineAngle*pi/180), Rr=ZoneImpedance(2)*cos(LineAngle*pi/180), Td=ZoneTime(2)}
      mask prompts: Xr "Reactance reach [ohm]"; Rr "Resistance reach [ohm]"; Td "Time delay [s]"
  Zone 3 : Subsystem  mask(Zone){Xr=ZoneImpedance(3)*sin(LineAngle*pi/180), Rr=ZoneImpedance(3)*cos(LineAngle*pi/180), Td=ZoneTime(3)}
      mask prompts: Xr "Reactance reach [ohm]"; Rr "Resistance reach [ohm]"; Td "Time delay [s]"
  Zone 4 : Subsystem  mask(Zone){Xr=ZoneImpedance(4)*sin(LineAngle*pi/180), Rr=ZoneImpedance(4)*cos(LineAngle*pi/180), Td=ZoneTime(4)}
      mask prompts: Xr "Reactance reach [ohm]"; Rr "Resistance reach [ohm]"; Td "Time delay [s]"
  Zone R : Subsystem  mask(Zone){Xr=ZoneImpedance(5)*sin(LineAngle*pi/180), Rr=ZoneImpedance(5)*cos(LineAngle*pi/180), Td=ZoneTime(5)}
      mask prompts: Xr "Reactance reach [ohm]"; Rr "Resistance reach [ohm]"; Td "Time delay [s]"
  Zone1Z : Terminator
  Zone2Z : Terminator
  Zone3Z : Terminator
  Zone4Z : Terminator
  ZoneRZ : Terminator
  Zone1 : Outport  InitialOutput=0
  Zone2 : Outport  Port=2  InitialOutput=0
  Zone3 : Outport  Port=3  InitialOutput=0
  Starter : Outport  Port=4  InitialOutput=0
  ZoneR : Outport  Port=5  InitialOutput=0
  "R, X" : Outport  Port=6  InitialOutput=0
  wires:
  Voltage Current/2 -> Impedance Module/2
  Voltage Current/1 -> Impedance Module/1
  Impedance Module/1 -> Complex to Real-Imag/1
  Mux4/1 -> Zone4Z/1
  Mux3/1 -> Zone3Z/1
  Mux2/1 -> Zone2Z/1
  Mux1/1 -> Zone1Z/1
  <V/1 -> Zone R/2(<V), Zone 4/2(<V), Zone 3/2(<V), Zone 2/2(<V), Zone 1/2(<V)
  Complex to Real-Imag/2 -> Mux6/2, Mux/2
  Complex to Real-Imag/1 -> Mux6/1, Mux/1
  Zone 4/1(TRIP) -> Starter/1
  Zone 3/1(TRIP) -> Zone3/1
  Zone 2/1(TRIP) -> Zone2/1
  Zone 4/3(Zr) -> Mux4/2
  Zone 4/2(Zm) -> Mux4/1
  Zone 3/3(Zr) -> Mux3/2
  Zone 3/2(Zm) -> Mux3/1
  Zone 2/3(Zr) -> Mux2/2
  Zone 2/2(Zm) -> Mux2/1
  Zone 1/3(Zr) -> Mux1/2
  Zone 1/2(Zm) -> Mux1/1
  Zone 1/1(TRIP) -> Zone1/1
  Mux/1 -> Zone 2/1(Z), Zone R/1(Z), Zone 4/1(Z), Zone 3/1(Z), Zone 1/1(Z)
  B-C/1 -> Voltage Current/1
  Zone R/2(Zm) -> Mux5/1
  Zone R/3(Zr) -> Mux5/2
  Mux5/1 -> ZoneRZ/1
  Zone R/1(TRIP) -> ZoneR/1
  Mux6/1 -> "R, X"/1

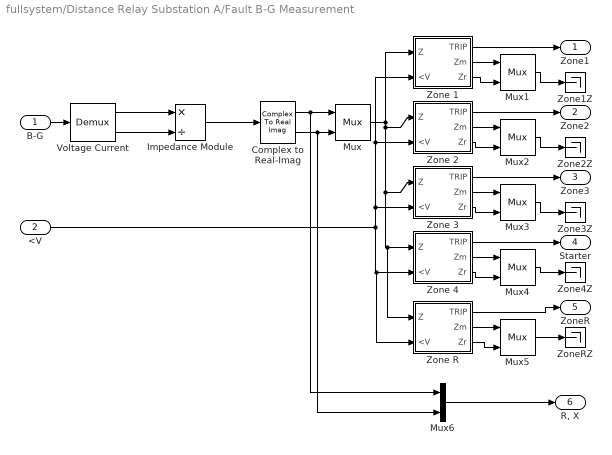
== system fullsystem/Distance Relay Substation A/Fault B-G Measurement ==
  B-G : Inport
  <V : Inport  Port=2
  Complex to Real-Imag : ComplexToRealImag
  Impedance Module : Product  Inputs=*/  SaturateOnIntegerOverflow=on  RndMeth=Zero  InputSameDT=on  OutDataTypeStr=Inherit: Same as first input
  Mux{,1..6} (7 alike) : Mux  Inputs=2
  Voltage Current : Demux  Outputs=2
  Zone 1 : Subsystem  mask(Zone){Xr=ZoneImpedance(1)*sin(LineAngle*pi/180), Rr=ZoneImpedance(1)*cos(LineAngle*pi/180), Td=ZoneTime(1)}
      mask prompts: Xr "Reactance reach [ohm]"; Rr "Resistance reach [ohm]"; Td "Time delay [s]"
  Zone 2 : Subsystem  mask(Zone){Xr=ZoneImpedance(2)*sin(LineAngle*pi/180), Rr=ZoneImpedance(2)*cos(LineAngle*pi/180), Td=ZoneTime(2)}
      mask prompts: Xr "Reactance reach [ohm]"; Rr "Resistance reach [ohm]"; Td "Time delay [s]"
  Zone 3 : Subsystem  mask(Zone){Xr=ZoneImpedance(3)*sin(LineAngle*pi/180), Rr=ZoneImpedance(3)*cos(LineAngle*pi/180), Td=ZoneTime(3)}
      mask prompts: Xr "Reactance reach [ohm]"; Rr "Resistance reach [ohm]"; Td "Time delay [s]"
  Zone 4 : Subsystem  mask(Zone){Xr=ZoneImpedance(4)*sin(LineAngle*pi/180), Rr=ZoneImpedance(4)*cos(LineAngle*pi/180), Td=ZoneTime(4)}
      mask prompts: Xr "Reactance reach [ohm]"; Rr "Resistance reach [ohm]"; Td "Time delay [s]"
  Zone R : Subsystem  mask(Zone){Xr=ZoneImpedance(5)*sin(LineAngle*pi/180), Rr=ZoneImpedance(5)*cos(LineAngle*pi/180), Td=ZoneTime(5)}
      mask prompts: Xr "Reactance reach [ohm]"; Rr "Resistance reach [ohm]"; Td "Time delay [s]"
  Zone1Z : Terminator
  Zone2Z : Terminator
  Zone3Z : Terminator
  Zone4Z : Terminator
  ZoneRZ : Terminator
  Zone1 : Outport  InitialOutput=0
  Zone2 : Outport  Port=2  InitialOutput=0
  Zone3 : Outport  Port=3  InitialOutput=0
  Starter : Outport  Port=4  InitialOutput=0
  ZoneR : Outport  Port=5  InitialOutput=0
  "R, X" : Outport  Port=6  InitialOutput=0
  wires:
  Voltage Current/2 -> Impedance Module/2
  Voltage Current/1 -> Impedance Module/1
  Impedance Module/1 -> Complex to Real-Imag/1
  Mux4/1 -> Zone4Z/1
  Mux3/1 -> Zone3Z/1
  Mux2/1 -> Zone2Z/1
  Mux1/1 -> Zone1Z/1
  <V/1 -> Zone R/2(<V), Zone 4/2(<V), Zone 3/2(<V), Zone 2/2(<V), Zone 1/2(<V)
  Complex to Real-Imag/2 -> Mux6/2, Mux/2
  Complex to Real-Imag/1 -> Mux6/1, Mux/1
  Zone 4/1(TRIP) -> Starter/1
  Zone 3/1(TRIP) -> Zone3/1
  Zone 2/1(TRIP) -> Zone2/1
  Zone 4/3(Zr) -> Mux4/2
  Zone 4/2(Zm) -> Mux4/1
  Zone 3/3(Zr) -> Mux3/2
  Zone 3/2(Zm) -> Mux3/1
  Zone 2/3(Zr) -> Mux2/2
  Zone 2/2(Zm) -> Mux2/1
  Zone 1/3(Zr) -> Mux1/2
  Zone 1/2(Zm) -> Mux1/1
  Zone 1/1(TRIP) -> Zone1/1
  Mux/1 -> Zone 2/1(Z), Zone R/1(Z), Zone 4/1(Z), Zone 3/1(Z), Zone 1/1(Z)
  B-G/1 -> Voltage Current/1
  Zone R/2(Zm) -> Mux5/1
  Zone R/3(Zr) -> Mux5/2
  Mux5/1 -> ZoneRZ/1
  Zone R/1(TRIP) -> ZoneR/1
  Mux6/1 -> "R, X"/1
